simulink model "regulator_LQR_comparison"  (Simulink 10.0)
settings: Solver=ode45  StartTime=0.0  StopTime=tsim  RelTol=1e-3  EnableMultiTasking=on
values from neighbouring files (symbols this model uses):
  C_states = eye(2)    [es2.m]
  D_states = [0 0]'    [es2.m]
  Klqr1 = lqr(A,B,Q,R)    [es2.m]
  sat_max = inf    [es2.m]
  sat_min = -inf    [es2.m]
  x0 = [0 10]    [es2.m]
undefined symbols (not defined in the file or in its folder): A, B, C, Klqr2
settings Model: Creator=Administrator  LastModifiedBy=Chiara
settings DataIOCC: LimitDataPoints=on  SignalLoggingSaveFormat=ModelDataLogs
settings OptimizationCC: ExpressionDepthLimit=2147483647  InitFltsAndDblsToZero=on
settings DebuggingCC: SolverPrmCheckMsg=warning  FcnCallInpInsideContextMsg=warning  StateNameClashWarn=warning
settings GRTTargetCC: GeneratePreprocessorConditionals=Disable all
settings ConfigComp: CovExternalEMLEnable=off  CovSFcnEnable=off

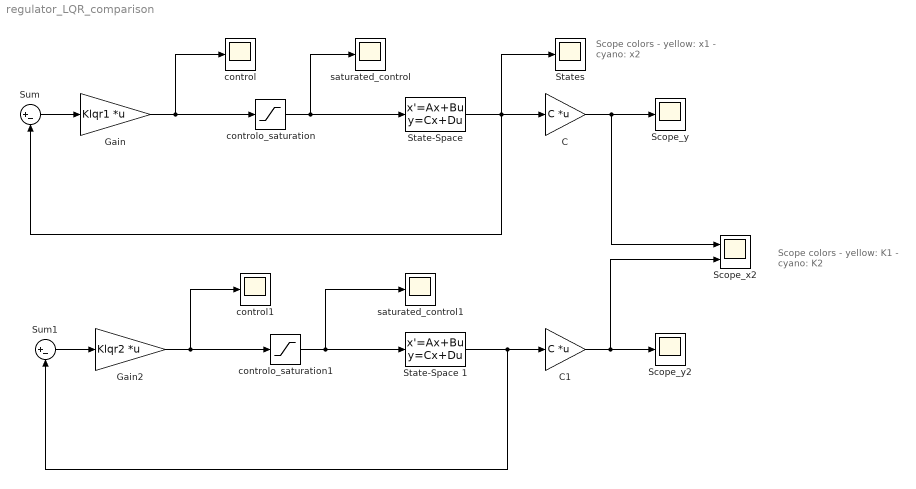
== system regulator_LQR_comparison ==
  note: Scope colors
      | - yellow: x1
      | - cyano: x2
  note: Scope colors
      | - yellow: K1
      | - cyano: K2
  C : Gain  Gain=C  Multiplication=Matrix(K*u)
  C1 : Gain  Gain=C  Multiplication=Matrix(K*u)
  Gain : Gain  Gain=Klqr1  Multiplication=Matrix(K*u)
  Gain2 : Gain  Gain=Klqr2  Multiplication=Matrix(K*u)
  Scope_x2 : Scope  NumInputPorts=2
  Scope_y : Scope
  Scope_y2 : Scope
  "State-Space " : StateSpace  A=A  B=B  C=C_states  D=D_states  InitialCondition=x0
  State-Space 1 : StateSpace  A=A  B=B  C=C_states  D=D_states  InitialCondition=x0
  States : Scope
  Sum : Sum  Inputs=|+-
  Sum1 : Sum  Inputs=|+-
  control : Scope
  control1 : Scope
  controlo_saturation : Saturate  UpperLimit=sat_max  LowerLimit=sat_min
  controlo_saturation1 : Saturate  UpperLimit=sat_max  LowerLimit=sat_min
  saturated_control : Scope
  saturated_control1 : Scope
  wires:
  controlo_saturation/1 -> "State-Space "/1, saturated_control/1
  Gain/1 -> controlo_saturation/1, control/1
  Sum/1 -> Gain/1
  "State-Space "/1 -> States/1, C/1, Sum/2
  State-Space 1/1 -> C1/1, Sum1/2
  Sum1/1 -> Gain2/1
  Gain2/1 -> controlo_saturation1/1, control1/1
  controlo_saturation1/1 -> State-Space 1/1, saturated_control1/1
  C/1 -> Scope_x2/1, Scope_y/1
  C1/1 -> Scope_x2/2, Scope_y2/1
